simulink model "simulacion_v1"  (R2021b)
settings: Solver=VariableStepAuto  StartTime=0.0  StopTime=100  RelTol=1e-3
undefined symbols (not defined in the file or in its folder): F, h, km, Light, m, MIL, Moderate, s, sigbuilder_block
libraries: slpidlib x19, simulink x18, simulink_extras x15, aerolibconvert2 x4, aerolibwind2 x3, shared6dof x1, sharedtransform x1, sim3dlib x1, uavsim3dlib x1
(part 3 of 3)

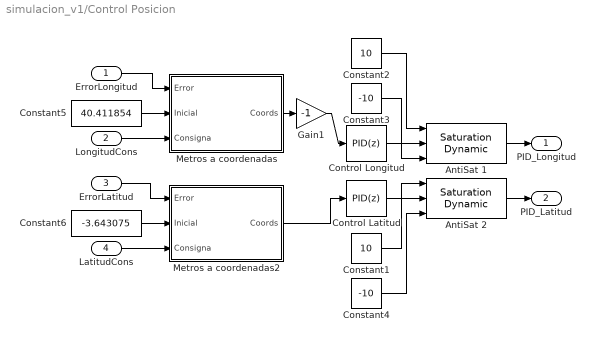
== system simulacion_v1/Control Posicion ==
  ErrorLongitud : Inport
  LongitudCons : Inport  Port=2
  ErrorLatitud : Inport  Port=3
  LatitudCons : Inport  Port=4
  AntiSat 1 : simulink/Discontinuities/Saturation Dynamic  OutMin=[]  OutMax=[]  OutDataTypeStr=Inherit: Same as second input  OutDataType=fixdt(1, 16)  OutScaling=2^-10  DoSatur=off
  AntiSat 2 : simulink/Discontinuities/Saturation Dynamic  OutMin=[]  OutMax=[]  OutDataTypeStr=Inherit: Same as second input  OutDataType=fixdt(1, 16)  OutScaling=2^-10  DoSatur=off
  Constant1 : Constant  Value=10
  Constant2 : Constant  Value=10
  Constant3 : Constant  Value=-10
  Constant4 : Constant  Value=-10
  Constant5 : Constant  Value=40.411854
  Constant6 : Constant  Value=-3.643075
  Control Latitud : slpidlib/PID Controller  Controller=PID  Form=Parallel  TimeDomain=Discrete-time  UseExternalTs=off  SampleTime=0.006  IntegratorMethod=Forward Euler  FilterMethod=Forward Euler  ControllerParametersSource=internal  P=1000000  I=10000  D=200000  UseFilter=off  N=100  TunerSelectOption=Transfer Function Based (PID Tuner App)  InitialConditionSource=internal  InitialConditionForIntegrator=0  InitialConditionForFilter=0  DifferentiatorICPrevScaledInput=0  ExternalReset=none  TrackingMode=off  Kt=1  LimitOutput=off  SatLimitsSource=internal  UpperSaturationLimit=inf  LowerSaturationLimit=-inf  LinearizeAsGain=off  AntiWindupMode=none  Kb=1  POutMin=[]  POutMax=[]  IOutMin=[]  IOutMax=[]  DOutMin=[]  DOutMax=[]  NOutMin=[]  NOutMax=[]  SumOutMin=[]  SumOutMax=[]  SaturationOutMin=[]  SaturationOutMax=[]  PParamMin=[]  PParamMax=[]  IParamMin=[]  IParamMax=[]  DParamMin=[]  DParamMax=[]  NParamMin=[]  NParamMax=[]  KbParamMin=[]  KbParamMax=[]  KtParamMin=[]  KtParamMax=[]  KbOutMin=[]  KbOutMax=[]  KtOutMin=[]  KtOutMax=[]  IntegratorOutMin=[]  IntegratorOutMax=[]  FilterOutMin=[]  FilterOutMax=[]  SumI1OutMin=[]  SumI1OutMax=[]  SumI2OutMin=[]  SumI2OutMax=[]  SumI3OutMin=[]  SumI3OutMax=[]  SumI4OutMin=[]  SumI4OutMax=[]  SumDOutMin=[]  SumDOutMax=[]  DifferentiatorOutMin=[]  DifferentiatorOutMax=[]  FilterDiffOutCoefMin=[]  FilterDiffOutCoefMax=[]  ReciprocalOutMin=[]  ReciprocalOutMax=[]  SumDenOutMin=[]  SumDenOutMax=[]  SumNumOutMin=[]  SumNumOutMax=[]  DivideOutMin=[]  DivideOutMax=[]  UdiffTsProdOutMin=[]  UdiffTsProdOutMax=[]  NTsProdOutMin=[]  NTsProdOutMax=[]  UintegralTsProdOutMin=[]  UintegralTsProdOutMax=[]  UngainTsProdOutMin=[]  UngainTsProdOutMax=[]  IntegratorContinuousStateAttributes=''  IntegratorStateMustResolveToSignalObject=off  IntegratorRTWStateStorageClass=Auto  FilterContinuousStateAttributes=''  FilterStateMustResolveToSignalObject=off  FilterRTWStateStorageClass=Auto  ParallelPVariant=InternalParameters  IdealPVariant=Disabled  IVariant=InternalParameters  DVariant=InternalParameters  IntegratorVariant=Discrete  SatVariant=Disabled  AWVariant=Passthrough  PCopyVariant=Disabled  TRVariant=Disabled  FdbkBlocksVariant=Forward  IdealPFdbkVariant=Disabled  SatFdbkVariant=Disabled  DerivativeFilterVariant=Differentiator  NVariant=Passthrough  NCopyVariant=Disabled_SignalSpec  FilterICVariant=InternalICsDifferentiator  IntegratorICVariant=InternalICs  ExternalResetVariant=Disabled  TRSumVariant=Passthrough  SumFdbkVariant=Disabled  SumVariant=Sum_PID  TsampFilterVariant=InternalTs  TsampNgainVariant=Passthrough  TsampIntegralVariant=Passthrough  ExternalSaturationOutDataTypeStr=Inherit: Same as second input
  Control Longitud : slpidlib/PID Controller  Controller=PID  Form=Parallel  TimeDomain=Discrete-time  UseExternalTs=off  SampleTime=0.006  IntegratorMethod=Forward Euler  FilterMethod=Forward Euler  ControllerParametersSource=internal  P=1000000  I=10000  D=200000  UseFilter=off  N=100  TunerSelectOption=Transfer Function Based (PID Tuner App)  InitialConditionSource=internal  InitialConditionForIntegrator=0  InitialConditionForFilter=0  DifferentiatorICPrevScaledInput=0  ExternalReset=none  TrackingMode=off  Kt=1  LimitOutput=off  SatLimitsSource=internal  UpperSaturationLimit=inf  LowerSaturationLimit=-inf  LinearizeAsGain=off  AntiWindupMode=none  Kb=1  POutMin=[]  POutMax=[]  IOutMin=[]  IOutMax=[]  DOutMin=[]  DOutMax=[]  NOutMin=[]  NOutMax=[]  SumOutMin=[]  SumOutMax=[]  SaturationOutMin=[]  SaturationOutMax=[]  PParamMin=[]  PParamMax=[]  IParamMin=[]  IParamMax=[]  DParamMin=[]  DParamMax=[]  NParamMin=[]  NParamMax=[]  KbParamMin=[]  KbParamMax=[]  KtParamMin=[]  KtParamMax=[]  KbOutMin=[]  KbOutMax=[]  KtOutMin=[]  KtOutMax=[]  IntegratorOutMin=[]  IntegratorOutMax=[]  FilterOutMin=[]  FilterOutMax=[]  SumI1OutMin=[]  SumI1OutMax=[]  SumI2OutMin=[]  SumI2OutMax=[]  SumI3OutMin=[]  SumI3OutMax=[]  SumI4OutMin=[]  SumI4OutMax=[]  SumDOutMin=[]  SumDOutMax=[]  DifferentiatorOutMin=[]  DifferentiatorOutMax=[]  FilterDiffOutCoefMin=[]  FilterDiffOutCoefMax=[]  ReciprocalOutMin=[]  ReciprocalOutMax=[]  SumDenOutMin=[]  SumDenOutMax=[]  SumNumOutMin=[]  SumNumOutMax=[]  DivideOutMin=[]  DivideOutMax=[]  UdiffTsProdOutMin=[]  UdiffTsProdOutMax=[]  NTsProdOutMin=[]  NTsProdOutMax=[]  UintegralTsProdOutMin=[]  UintegralTsProdOutMax=[]  UngainTsProdOutMin=[]  UngainTsProdOutMax=[]  IntegratorContinuousStateAttributes=''  IntegratorStateMustResolveToSignalObject=off  IntegratorRTWStateStorageClass=Auto  FilterContinuousStateAttributes=''  FilterStateMustResolveToSignalObject=off  FilterRTWStateStorageClass=Auto  ParallelPVariant=InternalParameters  IdealPVariant=Disabled  IVariant=InternalParameters  DVariant=InternalParameters  IntegratorVariant=Discrete  SatVariant=Disabled  AWVariant=Passthrough  PCopyVariant=Disabled  TRVariant=Disabled  FdbkBlocksVariant=Forward  IdealPFdbkVariant=Disabled  SatFdbkVariant=Disabled  DerivativeFilterVariant=Differentiator  NVariant=Passthrough  NCopyVariant=Disabled_SignalSpec  FilterICVariant=InternalICsDifferentiator  IntegratorICVariant=InternalICs  ExternalResetVariant=Disabled  TRSumVariant=Passthrough  SumFdbkVariant=Disabled  SumVariant=Sum_PID  TsampFilterVariant=InternalTs  TsampNgainVariant=Passthrough  TsampIntegralVariant=Passthrough  ExternalSaturationOutDataTypeStr=Inherit: Same as second input
  Gain1 : Gain  Gain=-1
  Metros a coordenadas : MATLAB Function  TreatAsAtomicUnit=on
  Metros a coordenadas2 : MATLAB Function  TreatAsAtomicUnit=on
  PID_Longitud : Outport
  PID_Latitud : Outport  Port=2
  wires:
  AntiSat 1/1 -> PID_Longitud/1
  Constant3/1 -> AntiSat 1/3
  Constant2/1 -> AntiSat 1/1
  Control Longitud/1 -> AntiSat 1/2
  Constant4/1 -> AntiSat 2/3
  Constant1/1 -> AntiSat 2/1
  Control Latitud/1 -> AntiSat 2/2
  AntiSat 2/1 -> PID_Latitud/1
  ErrorLongitud/1 -> Metros a coordenadas/1(Error)
  Constant5/1 -> Metros a coordenadas/2(Inicial)
  Metros a coordenadas/1(Coords) -> Gain1/1
  LongitudCons/1 -> Metros a coordenadas/3(Consigna)
  Gain1/1 -> Control Longitud/1
  Constant6/1 -> Metros a coordenadas2/2(Inicial)
  ErrorLatitud/1 -> Metros a coordenadas2/1(Error)
  LatitudCons/1 -> Metros a coordenadas2/3(Consigna)
  Metros a coordenadas2/1(Coords) -> Control Latitud/1

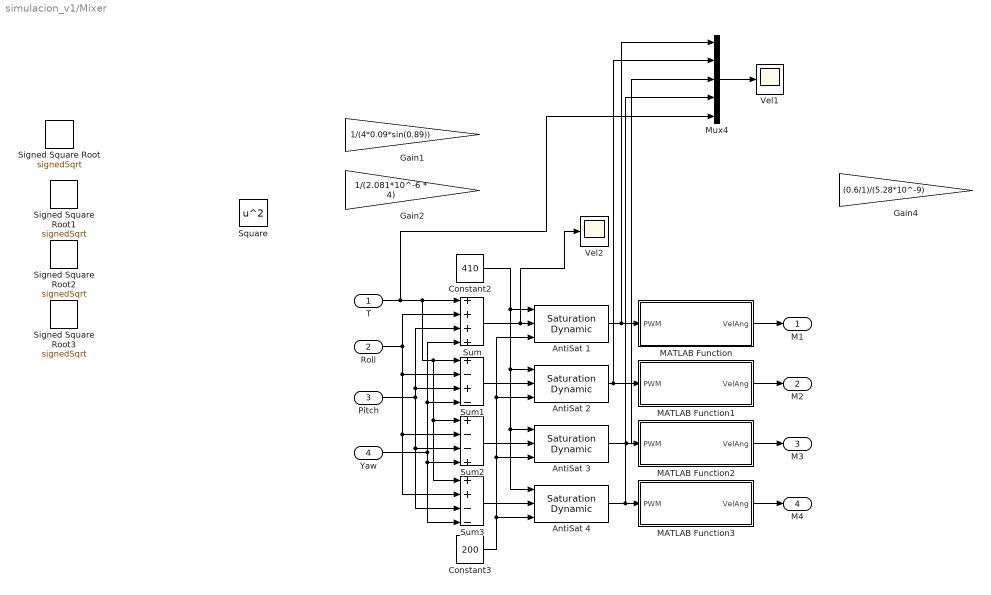
== system simulacion_v1/Mixer  ==
  T : Inport
  Roll : Inport  Port=2
  Pitch : Inport  Port=3
  Yaw : Inport  Port=4
  AntiSat {1..4} (4 alike) : simulink/Discontinuities/Saturation Dynamic  OutMin=[]  OutMax=[]  OutDataTypeStr=Inherit: Same as second input  OutDataType=fixdt(1, 16)  OutScaling=2^-10  DoSatur=off
  Constant2 : Constant  Value=410
  Constant3 : Constant  Value=200
  Gain1 : Gain  Gain=1/(4*0.09*sin(0.89))
  Gain2 : Gain  Gain=1/(2.081*10^-6 * 4)
  Gain4 : Gain  Gain=(0.6/1)/(5.28*10^-9)
  MATLAB Function : MATLAB Function  TreatAsAtomicUnit=on
  MATLAB Function1 : MATLAB Function  TreatAsAtomicUnit=on
  MATLAB Function2 : MATLAB Function  TreatAsAtomicUnit=on
  MATLAB Function3 : MATLAB Function  TreatAsAtomicUnit=on
  Mux4 : Mux  Inputs=5
  Signed Square Root{,1..3} (4 alike) : Sqrt  Operator=signedSqrt  SaturateOnIntegerOverflow=on
  Square : Math  Operator=square  SaturateOnIntegerOverflow=on
  Sum : Sum  Inputs=++++
  Sum1 : Sum  Inputs=+-+-
  Sum2 : Sum  Inputs=+--+
  Sum3 : Sum  Inputs=++--
  Vel1 : Scope
  Vel2 : Scope
  M1 : Outport
  "M2 " : Outport  Port=2
  M3 : Outport  Port=3
  M4 : Outport  Port=4
  wires:
  Roll/1 -> Sum3/2, Sum2/2, Sum1/2, Sum/2
  Pitch/1 -> Sum3/3, Sum2/3, Sum/3, Sum1/3
  Yaw/1 -> Sum3/4, Sum2/4, Sum/4, Sum1/4
  T/1 -> Mux4/5, Sum3/1, Sum2/1, Sum1/1, Sum/1
  AntiSat 1/1 -> Mux4/1, MATLAB Function/1(PWM)
  Constant2/1 -> AntiSat 1/1, AntiSat 2/1, AntiSat 3/1, AntiSat 4/1
  Sum/1 -> Vel2/1, AntiSat 1/2
  Sum1/1 -> AntiSat 2/2
  Sum2/1 -> AntiSat 3/2
  Sum3/1 -> AntiSat 4/2
  Constant3/1 -> AntiSat 4/3, AntiSat 3/3, AntiSat 1/3, AntiSat 2/3
  MATLAB Function2/1(VelAng) -> M3/1
  MATLAB Function1/1(VelAng) -> "M2 "/1
  MATLAB Function/1(VelAng) -> M1/1
  MATLAB Function3/1(VelAng) -> M4/1
  Mux4/1 -> Vel1/1
  AntiSat 3/1 -> Mux4/3, MATLAB Function2/1(PWM)
  AntiSat 4/1 -> Mux4/4, MATLAB Function3/1(PWM)
  AntiSat 2/1 -> Mux4/2, MATLAB Function1/1(PWM)

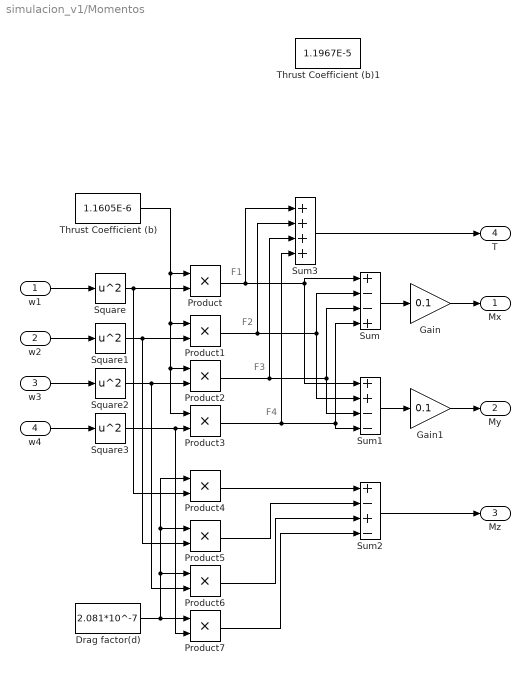
== system simulacion_v1/Momentos ==
  note: F4
  note: F3
  note: F2
  note: F1
  w1 : Inport
  w2 : Inport  Port=2
  w3 : Inport  Port=3
  w4 : Inport  Port=4
  Drag factor(d) : Constant  Value=2.081*10^-7
  Gain : Gain  Gain=0.1
  Gain1 : Gain  Gain=0.1
  Product{,1..7} (8 alike) : Product
  Square{,1..3} (4 alike) : Math  Operator=square  SaturateOnIntegerOverflow=on
  Sum : Sum  Inputs=+--+
  Sum1 : Sum  Inputs=++--
  Sum2 : Sum  Inputs=+-+-
  Sum3 : Sum  Inputs=++++
  Thrust Coefficient (b) : Constant  Value=1.1605E-6
  Thrust Coefficient (b)1 : Constant  Value=1.1967E-5
  Mx : Outport
  "My " : Outport  Port=2
  "Mz " : Outport  Port=3
  T : Outport  Port=4
  wires:
  Sum1/1 -> Gain1/1
  Product1/1 -> Sum/2, Sum1/2, Sum3/2
  Product/1 -> Sum1/1, Sum/1, Sum3/1
  Product2/1 -> Sum1/3, Sum/3, Sum3/3
  Product3/1 -> Sum/4, Sum1/4, Sum3/4
  Gain1/1 -> "My "/1
  Gain/1 -> Mx/1
  Sum/1 -> Gain/1
  Sum2/1 -> "Mz "/1
  Square3/1 -> Product7/2, Product3/2
  Square1/1 -> Product1/2, Product5/2
  Thrust Coefficient (b)/1 -> Product3/1, Product2/1, Product1/1, Product/1
  Square2/1 -> Product2/2, Product6/2
  Square/1 -> Product/2, Product4/2
  Drag factor(d)/1 -> Product4/1, Product5/1, Product6/1, Product7/1
  Product4/1 -> Sum2/1
  Product5/1 -> Sum2/2
  Product6/1 -> Sum2/3
  Sum3/1 -> T/1
  w1/1 -> Square/1
  w2/1 -> Square1/1
  w3/1 -> Square2/1
  w4/1 -> Square3/1
  Product7/1 -> Sum2/4

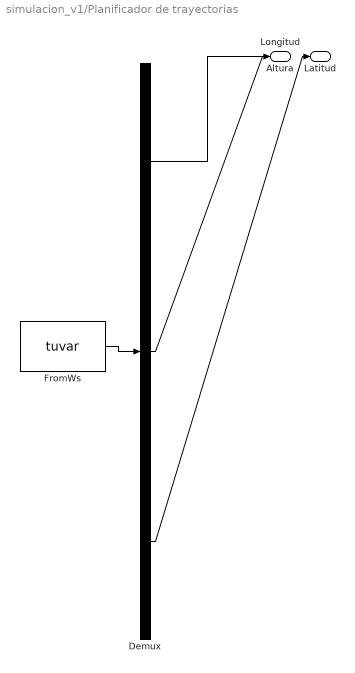
== system simulacion_v1/Planificador de trayectorias ==
  Demux : Demux  Tag=STV Demux  Outputs=3
      settings: DisplayOption=none
  FromWs : FromWorkspace  Tag=STV FromWs  VariableName=tuvar
      SigBuilderData=|
      | common.afterFinalStr = 'Extrapolate'
      | common.sampleTime = 0
      | dataSet.timeRange = [0 100]
      | dataSet.name = 'Señales Modo Autonomo'
      | sbobj.Groups.Name = 'Señales Modo Autonomo'
      | sbobj.Groups.Signals(1).Name = 'Altura'
      | sbobj.Groups.Signals(1).XData = [0 100]
      | sbobj.Groups.Signals(1).YData = [5 5]
      | sbobj.Groups.Signals(2).Name = 'Longitud'
      | sbobj.Groups.Signals(2).XData = [0 46 50 80 100]
      | sbobj.Groups.Signals(2).YData = [0 0 0 0 0]
      | sbobj.Groups.Signals(3).Name = 'Latitud'
      | sbobj.Groups.Signals(3).XData = [0 46 64.5 70 100]
      | sbobj.Groups.Signals(3).YData = [0 0 0 0 0]
      | sbobj.Groups.TimeRange = [0 100]
  Altura : Outport  Tag=STV Outport
  Longitud : Outport  Tag=STV Outport  Port=2
  Latitud : Outport  Tag=STV Outport  Port=3
  wires:
  FromWs/1 -> Demux/1
  Demux/1 -> Altura/1
  Demux/2 -> Longitud/1
  Demux/3 -> Latitud/1

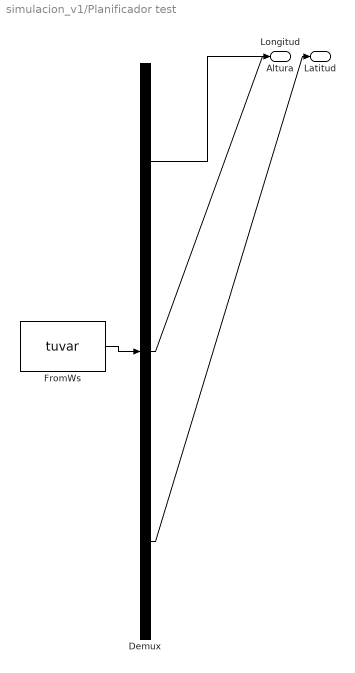
== system simulacion_v1/Planificador test ==
  Demux : Demux  Tag=STV Demux  Outputs=3
      settings: DisplayOption=none
  FromWs : FromWorkspace  Tag=STV FromWs  VariableName=tuvar
      SigBuilderData=|
      | common.afterFinalStr = 'Extrapolate'
      | common.sampleTime = 0
      | dataSet.timeRange = [0 100]
      | dataSet.name = 'Señales Modo Autonomo'
      | sbobj.Groups.Name = 'Señales Modo Autonomo'
      | sbobj.Groups.Signals(1).Name = 'Altura'
      | sbobj.Groups.Signals(1).XData = [0 100]
      | sbobj.Groups.Signals(1).YData = [5 5]
      | sbobj.Groups.Signals(2).Name = 'Longitud'
      | sbobj.Groups.Signals(2).XData = [0 10 10 25 50 50 80 100]
      | sbobj.Groups.Signals(2).YData = [0 0 -10 -10 -10 0 0 0]
      | sbobj.Groups.Signals(3).Name = 'Latitud'
      | sbobj.Groups.Signals(3).XData = [0 25 25 65 65 100]
      | sbobj.Groups.Signals(3).YData = [0 0 -10 -10 0 0]
      | sbobj.Groups.TimeRange = [0 100]
  Altura : Outport  Tag=STV Outport
  Longitud : Outport  Tag=STV Outport  Port=2
  Latitud : Outport  Tag=STV Outport  Port=3
  wires:
  FromWs/1 -> Demux/1
  Demux/1 -> Altura/1
  Demux/2 -> Longitud/1
  Demux/3 -> Latitud/1

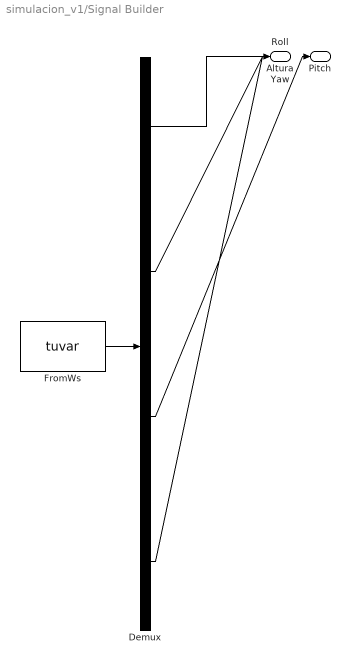
== system simulacion_v1/Signal Builder ==
  Demux : Demux  Tag=STV Demux
      settings: DisplayOption=none
  FromWs : FromWorkspace  Tag=STV FromWs  VariableName=tuvar
      SigBuilderData=|
      | common.afterFinalStr = 'Extrapolate'
      | common.sampleTime = 0
      | dataSet.timeRange = [0 100]
      | dataSet.name = 'Señales Modo Manual'
      | sbobj.Groups.Name = 'Señales Modo Manual'
      | sbobj.Groups.Signals(1).Name = 'Altura'
      | sbobj.Groups.Signals(1).XData = [0 90 100]
      | sbobj.Groups.Signals(1).YData = [5 5 5]
      | sbobj.Groups.Signals(2).Name = 'Roll'
      | sbobj.Groups.Signals(2).XData = [0 20 20 30 30 40 40 50 50 100]
      | sbobj.Groups.Signals(2).YData = [0 0 15 15 0 0 -15 -15 0 0]
      | sbobj.Groups.Signals(3).Name = 'Pitch'
      | sbobj.Groups.Signals(3).XData = [0 60 60 70 70 80 80 90 90 100]
      | sbobj.Groups.Signals(3).YData = [0 0 15 15 0 0 -15 -15 0 0]
      | sbobj.Groups.Signals(4).Name = 'Yaw'
      | sbobj.Groups.Signals(4).XData = [0 100]
      | sbobj.Groups.Signals(4).YData = [0 0]
      | sbobj.Groups.TimeRange = [0 100]
  Altura : Outport  Tag=STV Outport
  Roll : Outport  Tag=STV Outport  Port=2
  Pitch : Outport  Tag=STV Outport  Port=3
  Yaw : Outport  Tag=STV Outport  Port=4
  wires:
  FromWs/1 -> Demux/1
  Demux/1 -> Altura/1
  Demux/2 -> Roll/1
  Demux/3 -> Pitch/1
  Demux/4 -> Yaw/1

== matlab function simulacion_v1/Mixer /MATLAB Function ==
  data: PWM input; VelAng output
function VelAng = PWM_to_VelAng(PWM)

VelAng =-0.0124*PWM^2+16.697*PWM-2842.4;

== matlab function simulacion_v1/MATLAB Function ==
  data: u input; F_earth output; c input; mass input; h input; v input
function F_earth = fcn(u,c,mass,h,v)
phi = u(1);
theta = u(2);
psi = u(3);

Rx = [1 0 0; 0 cos(phi) -sin(phi); 0 sin(phi) cos(phi)];
Ry = [cos(theta) 0 sin(theta); 0 1 0;-sin(theta) 0 cos(theta)];
Rz = [cos(psi) -sin(psi) 0; sin(psi) cos(psi) 0; 0 0 1];

R = Rz*Ry*Rx;

v_r = v'*R;
vx = v_r(1);
vy = v_r(2);
vz = v_r(3);

g = 9.81;

% Rozamiento lineal
A_r = 0.435;
A_rz = 0.01;

Zx = vx * A_r;
Zy = vy * A_r;
Zz = vz * A_rz;


FORCES = mass*[0 0 g]' - R*[0 0 c]' - [Zx Zy Zz]';

% if h <= 0
%     if v > 0
%         FORCES(3,1) = - mass * (v/0.00001);
%     elseif v == 0
%         FORCES = mass*[0 0 0]' - R*[0 0 c]';
%     elseif v <= 0
%         FORCES = mass*[0 0 g]' - R*[0 0 c]';
%     end   
% end

F_earth = FORCES;

== matlab function simulacion_v1/Mixer /MATLAB Function1 ==
  data: PWM input; VelAng output
function VelAng = PWM_to_VelAng(PWM)

VelAng =-0.0124*PWM^2+16.697*PWM-2842.4;

== matlab function simulacion_v1/Mixer /MATLAB Function2 ==
  data: PWM input; VelAng output
function VelAng = PWM_to_VelAng(PWM)

VelAng =-0.0124*PWM^2+16.697*PWM-2842.4;

== matlab function simulacion_v1/Mixer /MATLAB Function3 ==
  data: PWM input; VelAng output
function VelAng = PWM_to_VelAng(PWM)
VelAng =-0.0124*PWM^2+16.697*PWM-2842.4;

== matlab function simulacion_v1/MATLAB Function1 ==
  data: u input; y output
function y = fcn(u)

y = sqrt(u(1)^2+u(2)^2);

== matlab function simulacion_v1/Control Posicion/Metros a coordenadas2 ==
  data: Error input; Coords output; Inicial input; Consigna input
% function Coords = fcn(Error, Inicial, Consigna, Inicial_Lat, Consigna_Lat)
% 
% Coordenada_home_lat = 40.411854;
% Coordenada_home_long = -3.643075;
% 
% Latconsigna = (180 / pi) * (Inicial_Lat * (pi / 180) + Consigna_Lat / 6372795);
% 
% if Error < 0
% Coordsconsigna = (180 / pi) * (Inicial * (pi / 180) - acos((cos(Consigna / 6372795) - (sin(Latconsigna * (pi / 180)))^2 / ((cos(Latconsigna * (pi / 180)))^2))));
% else
% Coordsconsigna = (180 / pi) * (Inicial * (pi / 180) + acos((cos(Consigna / 6372795) - (sin(Latconsigna * (pi / 180)))^2 / ((cos(Latconsigna * (pi / 180)))^2))));
% end
% 
% if Error < 0
% Coordsactuales = (180 / pi) * (Coordsconsigna * (pi / 180) - acos((cos(Error / 6372795) - (sin(Latconsigna * (pi / 180)))^2 / ((cos(Latconsigna * (pi / 180)))^2))));
% else
% Coordsactuales = (180 / pi) * (Coordsconsigna * (pi / 180) + acos((cos(Error / 6372795) - (sin(Latconsigna * (pi / 180)))^2 / ((cos(Latconsigna * (pi / 180)))^2))));
% end
% 
% Coords = Coordsconsigna - Coordsactuales;


function Coords = fcn(Error, Inicial, Consigna)

Coordenada_home_lat = 40.411854;
Coordenada_home_long = -3.643075;

Coordsconsigna = (180 / pi) * (Inicial * (pi / 180) + Consigna / 6372795);

Coordsactuales = (180 / pi) * (Coordsconsigna * (pi / 180) + Error / 6372795);

Coords = Coordsconsigna - Coordsactuales;

== matlab function simulacion_v1/Control Posicion/Metros a coordenadas ==
  data: Error input; Coords output; Inicial input; Consigna input
function Coords = fcn(Error, Inicial, Consigna)

Coordenada_home_lat = 40.411854;
Coordenada_home_long = -3.643075;

Coordsconsigna = (180 / pi) * (Inicial * (pi / 180) + Consigna / 6372795);

Coordsactuales = (180 / pi) * (Coordsconsigna * (pi / 180) + Error / 6372795);

Coords = Coordsconsigna - Coordsactuales;
